simulink model "flightControlSystem"  (R2020b)
settings: Solver=ode3  StartTime=0  StopTime=inf  FixedStep=Ts  RelTol=1e-3  EnableMultiTasking=on
model workspace (MAT data in the model file):
  bwmaskcircle : Simulink.Parameter (value not decoded)
  bwmaskcorner : Simulink.Parameter (value not decoded)
  bwmaskland : Simulink.Parameter (value not decoded)
  bwmaskleft : Simulink.Parameter (value not decoded)
  bwmaskleftmatrix = [0 0 0 0 0 0 0 0 0 0 0 0 ... (6912000 elements, 120x160x360)]
  bwmaskpathtrianglematrix = [0 0 0 0 0 0 0 0 0 0 0 0 ... (6931200 elements, 120x160x361)]
  bwmaskpathtrianglematrix360 = [0 0 0 0 0 0 0 0 0 0 0 0 ... (6912000 elements, 120x160x360)]
  bwmaskright : Simulink.Parameter (value not decoded)
  bwmaskrightmatrix = [0 0 0 0 0 0 0 0 0 0 0 0 ... (6912000 elements, 120x160x360)]
  bwmasksquare : Simulink.Parameter (value not decoded)
  bwmasktrapezoid : Simulink.Parameter (value not decoded)
  bwmasktrapezoidmatrix = [0 0 0 0 0 0 0 0 0 0 0 0 ... (6931200 elements, 120x160x361)]
  bwmasktrapezoidmatrix360 = [0 0 0 0 0 0 0 0 0 0 0 0 ... (6912000 elements, 120x160x360)]
  bwmasktrapezoidmatrixold = [0 0 0 0 0 0 0 0 0 0 0 0 ... (6912000 elements, 120x160x360)]
  bwmasktraveled : Simulink.Parameter (value not decoded)
  bwmasktraveledmatrix = [1 1 1 1 1 1 1 1 1 1 1 1 ... (6931200 elements, 120x160x361)]
  bwmasktraveledmatrix360 = [0 0 0 0 0 0 0 0 0 0 0 0 ... (6912000 elements, 120x160x360)]
  bwmasktraveledpast : Simulink.Parameter (value not decoded)
symbols that are objects in the model workspace (value not decoded): bwmaskcircle
undefined symbols (not defined in the file): bwmaskpathtrianglematrixmatlab, bwmasktrapezoidmatrixmatlab, bwmasktraveledmatrixmatlab, codertarget, Controller, DiscIntNeverNeededParam, Discrete, Estimator, g, gray, init, orient_ref, pos_ref, Sensors, strel, Time, Ts, var_acc_angle_N, var_bias_gyr_N, var_gyro_p_N, Vehicle
libraries: simulink x40, pid_lib x5, ctrlSharedLib x4, sharedtransform x3, visiontextngfix x3, visionstatistics x2, visionmorphops x2, parrotlib x1, simulink_extras x1
(part 4 of 4)

== system flightControlSystem/Control System/State Estimator/XY Position Estimator/EstimatorVelocity/xy velocity w//o angular velocity compensation ==
  note: Optical flow raw readings are converted to velocity in m/s based on the estimated altitude
  optical_flow : Inport
  z_estimate : Inport  Port=2
  " " : Product  Inputs=**
  Compare To Constant : simulink/Logic and Bit Operations/Compare To Constant  relop=<  const=200*4  OutDataTypeStr=boolean
  Counter Free-Running : simulink/Sources/Counter Free-Running  NumBits=32  tsamp=-1
  Gain : Gain  Gain=-1
  Select dxy : Selector  InputPortWidth=3  IndexOptions=Index vector (dialog)  Indices=[1 2]  OutputSizes=1
  Switch : Switch  Criteria=u2 > Threshold
  opticalFlowErrorCorrect : Gain  Gain=1.15
  optical_flow_dx_dy : Outport
  wires:
  Select dxy/1 -> optical_flow_dx_dy/1  "optical_flow_dx_dy"
  " "/1 -> opticalFlowErrorCorrect/1
  opticalFlowErrorCorrect/1 -> Switch/3
  Gain/1 -> " "/2
  Switch/1 -> Select dxy/1
  Counter Free-Running/1 -> Compare To Constant/1
  Compare To Constant/1 -> Switch/2
  optical_flow/1 -> " "/1, Switch/1
  z_estimate/1 -> Gain/1

== matlab function flightControlSystem/Image Processing System/MATLAB Function2 ==
  data: bwmaskpathboolean input; bwmaskpathtriangle input; dHeading output
function dHeading  = fcn(bwmaskpathboolean, bwmaskpathtriangle)
bwmaskpathboolean = int8(bwmaskpathboolean);
bwmaskpathtriangleboolean = bwmaskpathboolean.*bwmaskpathtriangle;
sumDiff = sum(bwmaskpathtriangleboolean,'all');

%sumRight = sum(bwmaskright, 'all');
%sumLeft = sum(bwmaskleft, 'all');
%sumDiff = sumRight - sumLeft;
dHeading = 0.001*sumDiff;

== matlab function flightControlSystem/Image Processing System/MATLAB Function10 ==
  data: bwmaskcircle input; headingRefTOFlag output; bwmasktraveled input; noNextHeadingCornerFlag output
function [headingRefTOFlag, noNextHeadingCornerFlag]= fcn(bwmaskcircle, bwmasktraveled)
sumMatrix = sum(bwmaskcircle,'all');
sumTraveled = sum(bwmasktraveled,'all');
if sumMatrix < 5
    headingRefTOFlag = true;
else
    headingRefTOFlag = false;
end

if sumTraveled < 5
    noNextHeadingCornerFlag = true;
else
    noNextHeadingCornerFlag = false;
end

end

== stateflow chart flightControlSystem/Control System/Path Planning/Chart ==
  state wait [commented out]
    entry:
    xOut = single(0);
    yOut = single(0);
    zOut = zEstim;
  state takeoff
    entry:
    xOut = single(0);
    yOut = single(0);
    zOut = - 1;
    yawRef = 0;
  state flight
    during:
    xOut = xEstim + speed*cos(headingRef)
    yOut = yEstim + speed*sin(headingRef)
  state finish
    entry:
    xOut = xEstim;
    yOut = yEstim;
    zOut = 0;
  state land
    during:
    xOut = xEstim;
    yOut = yEstim;
    zOut = zEstim + 0.1;
  wait -> flight [commented out] : [after(2,sec)]
  takeoff -> wait [commented out] : [zEstim <= -1]
  (default) -> takeoff
  takeoff -> flight : [zEstim<=-1]
  flight -> land : [landNow == 1]
  land -> finish : [zOut > -0.5]
  data: xEstim input; yEstim input; zEstim input double; xOut output; yOut output; zOut output double; yawRef output single; yawEstim input; landNow input single; headingRef input; speed input single

== matlab function flightControlSystem/Control System/Path Planning/MATLAB Function1 ==
  data: yaw input; centroid input; x output; x_prev input; y output; y_prev input
function [x,y] = fcn(yaw, centroid, x_prev, y_prev)
    x = x_prev + 0.0005*cos(yaw);
    y = y_prev + 0.0005*sin(yaw) - 0.1*centroid(2);

== matlab function flightControlSystem/Image Processing System/landNow/landNow ==
  data: landNow output; centroidShifted input; majorAxis input; minorAxis input; ecc input; ext input
function landNow   = fcn(centroidShifted, majorAxis, minorAxis, ecc, ext)
% width = boundingBox(3);
% height = boundingBox(4);
% AR = width/height;
% diff = abs(AR - 1);
%  dx = centroidShifted(1);
%  dy = centroidShifted(2);
%  if (dx < 1 && dy < 5)
%      centroidNear = 1;
%      else
%      centroidNear = 0;
%  end
% if (diff < 0.2 && blobJumpFlag == 1 && centroidNear == 1)
%     landNow = 1;
% else
%     landNow = 0;
% end
% end

AR = minorAxis/majorAxis;
diff = abs(AR - 1);
eccFlag = (ecc < 0.25);
extFlag = (ext>0.6) && (ext<0.9);
dx = centroidShifted(1);
dy = centroidShifted(2);
if (abs(dx) < 5 && abs(dy) < 5)
    centroidNear = true;
else
    centroidNear = false;
end
 
 
if (diff < 0.2 && centroidNear == true && eccFlag == true && extFlag == true)
    landNow = 1;
else
    landNow = 0;
end

end

== matlab function flightControlSystem/Image Processing System/MATLAB Function4 ==
  data: centroidShifted input; cornerHeadingRef output
function cornerHeadingRef = fcn(centroidShifted)
    dx = centroidShifted(1);
    dy = centroidShifted(2);
    cornerHeadingRef = atan2(dx,dy);

== matlab function flightControlSystem/Image Processing System/MATLAB Function3 ==
  data: I input; Iangled output; angle input
function Iangled = fcn(I, angle)
i = angle + 181;
Iangled = I(:,:,i);
end

== matlab function flightControlSystem/Image Processing System/MATLAB Function6 ==
  data: angle input; wrappedAngle output
function wrappedAngle = fcn(angle)
if angle > 180
    wrappedAngle = angle - 360;
elseif angle < -180
    wrappedAngle = angle + 360;
else
    wrappedAngle = angle;
end

== matlab function flightControlSystem/Image Processing System/MATLAB Function5 ==
  data: bwmasktrapezoid input; majorHeadingChange output; sumtrapezoid output; speed output
function [majorHeadingChange, sumtrapezoid, speed] = fcn(bwmasktrapezoid)
sumtrapezoid = sum(bwmasktrapezoid, 'all');

%speed = 0.1 + (sumtrapezoid/850)*0.2
speed = 0.3*exp(-0.015*(800-sumtrapezoid)) + 0.15;

if sumtrapezoid < 5
    majorHeadingChange = true;
else
    majorHeadingChange = false;
end
end

== matlab function flightControlSystem/Image Processing System/landNow/MATLAB Function7 ==
  data: centroid input; centroidShifted output
function centroidShifted = fcn(centroid)
    dx = centroid(1)- 80;
    dy = 60 - centroid(2);
    centroidShifted = [dx, dy]

== matlab function flightControlSystem/Image Processing System/MATLAB Function8 ==
  data: majorHeadingChange input; cornerHeadingRef input; headingRef output; headingRefPrev input; dHeading input; pts output; headingRefTOFlag input; noNextHeadingCornerFlag input
function [headingRef, pts] = fcn(majorHeadingChange, cornerHeadingRef, headingRefPrev, dHeading, headingRefTOFlag, noNextHeadingCornerFlag)
if majorHeadingChange == true
    if noNextHeadingCornerFlag == true
    headingRef = headingRefPrev;    
    else
    headingRef = cornerHeadingRef;
    end
else
    headingRef = headingRefPrev + dHeading;
end

if headingRefTOFlag == true
    headingRef = headingRefPrev;
end

x1 = 0;
y1 = 0;
x2 = 30*cos(-headingRef+pi/2);
y2 = 30*sin(-headingRef+pi/2);

x1 = x1 + 80;
x2 = x2 + 80;
y1 = 60 - y1;
y2 = 60 - y2;
pts = [x1, y1, x2, y2];

== matlab function flightControlSystem/Image Processing System/MATLAB Function7 ==
  data: I input; Iangled output; angle input
function Iangled = fcn(I, angle)
i = angle + 181;
Iangled = I(:,:,i);
end

== matlab function flightControlSystem/Image Processing System/MATLAB Function9 ==
  data: I input; Iangled output; angle input
function Iangled = fcn(I, angle)
i = angle + 181;
Iangled = I(:,:,i);
end

== matlab function flightControlSystem/Image Processing System/MATLAB Function ==
  data: R input; BW output; G input; B input
function BW  = createMask(R, G, B)
%createMask  Threshold RGB image using auto-generated code from colorThresholder app.
%  [BW,MASKEDRGBIMAGE] = createMask(RGB) thresholds image RGB using
%  auto-generated code from the colorThresholder app. The colorspace and
%  range for each channel of the colorspace were set within the app. The
%  segmentation mask is returned in BW, and a composite of the mask and
%  original RGB images is returned in maskedRGBImage.

% Auto-generated by colorThresholder app on 16-Mar-2021
%------------------------------------------------------


% Convert RGB image to chosen color space


% Define thresholds for channel 1 based on histogram settings
channel1Min = 100.000;
channel1Max = 255.000;

% Define thresholds for channel 2 based on histogram settings
channel2Min = 0.000;
channel2Max = 128.000;

% Define thresholds for channel 3 based on histogram settings
channel3Min = 0.000;
channel3Max = 128.000;

% Create mask based on chosen histogram thresholds
sliderBW = (R >= channel1Min ) & (R <= channel1Max) & ...
    (G >= channel2Min ) & (G <= channel2Max) & ...
    (B >= channel3Min ) & (B <= channel3Max);
BW = sliderBW;


end

== matlab function flightControlSystem/Control System/Controller/Position Controller/Position error transformation (Earth to Body frame) ==
  data: yaw input; xy_err_earth input; xy_err_body output
function xy_err_body = fcn(yaw,xy_err_earth)

transformation = [cos(yaw), sin(yaw); -sin(yaw),  cos(yaw)];
xy_err_body = transformation * xy_err_earth;


end

== matlab function flightControlSystem/Image Processing System/MATLAB Function1 ==
  data: centroid input; centroidShifted output
function centroidShifted  = fcn(centroid)
dx = centroid(1)- 80;
dy = 60 - centroid(2);
centroidShifted = [dx, dy];
end
